simulink model "Oving4Oppg5b"  (R2020b)
settings: Solver=VariableStepAuto  StartTime=0.0  StopTime=130  MaxStep=0.01  RelTol=1e-3
values from neighbouring files (symbols this model uses):
  A = 2.34    [Oving4Oppg5Variables.mat]
  C_d = 0.24    [Oving4Oppg5Variables.mat]
  d = -3696.57031172    [Oving4Oppg5Variables.mat]
  k_F = 17.199    [Oving4Oppg5Variables.mat]
  k_P = 4322.801    [Oving4Oppg5Variables.mat]
  m = 2170    [Oving4Oppg5Variables.mat]
  rho = 1.225    [Oving4Oppg5Variables.mat]
  u_0 = -214.9875    [Oving4Oppg5Variables.mat]
  v_0 = 25    [Oving4Oppg5Variables.mat]
settings Model: Creator=crezl  LastModifiedBy=crezl

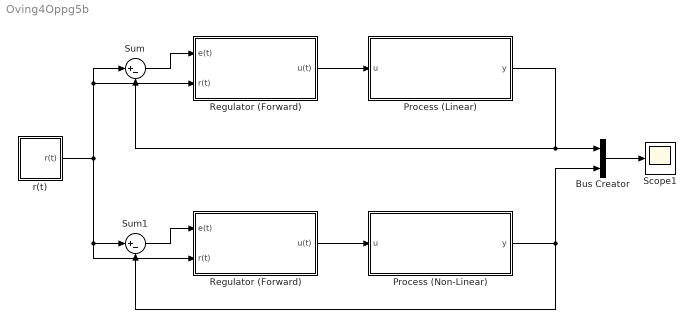
== system Oving4Oppg5b ==
  Bus Creator : BusCreator  Inputs=2
  Process (Linear) : Subsystem
  Process (Non-Linear) : Subsystem
  Regulator (Forward) : Subsystem
  "Regulator (Forward) " : Subsystem
  Scope1 : Scope
  Sum : Sum  Inputs=|+-
  Sum1 : Sum  Inputs=|+-
  r(t) : Subsystem
  wires:
  Process (Linear)/1(y) -> Sum/2, Bus Creator/1
  Bus Creator/1 -> Scope1/1
  Process (Non-Linear)/1(y) -> Bus Creator/2, Sum1/2
  Sum/1 -> Regulator (Forward)/1(e(t))
  r(t)/1(r(t)) -> "Regulator (Forward) "/2(r(t)), Sum1/1, Regulator (Forward)/2(r(t)), Sum/1
  Regulator (Forward)/1(u(t)) -> Process (Linear)/1(u)
  "Regulator (Forward) "/1(u(t)) -> Process (Non-Linear)/1(u)
  Sum1/1 -> "Regulator (Forward) "/1(e(t))

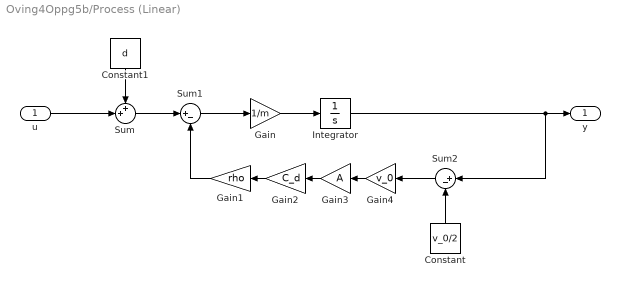
== system Oving4Oppg5b/Process (Linear) ==
  u : Inport
  Constant : Constant  Value=v_0/2
  Constant1 : Constant  Value=d
  Gain : Gain  Gain=1/m
  Gain1 : Gain  Gain=rho
  Gain2 : Gain  Gain=C_d
  Gain3 : Gain  Gain=A
  Gain4 : Gain  Gain=v_0
  Integrator : Integrator  InitialCondition=v_0
  Sum : Sum  Inputs=++|
  Sum1 : Sum  Inputs=|+-
  Sum2 : Sum  Inputs=|+-
  y : Outport
  wires:
  Constant1/1 -> Sum/1
  Integrator/1 -> Sum2/1, y/1
  Sum/1 -> Sum1/1
  Gain1/1 -> Sum1/2
  Sum1/1 -> Gain/1
  Gain3/1 -> Gain2/1
  Gain2/1 -> Gain1/1
  Gain/1 -> Integrator/1
  u/1 -> Sum/2
  Gain4/1 -> Gain3/1
  Constant/1 -> Sum2/2
  Sum2/1 -> Gain4/1

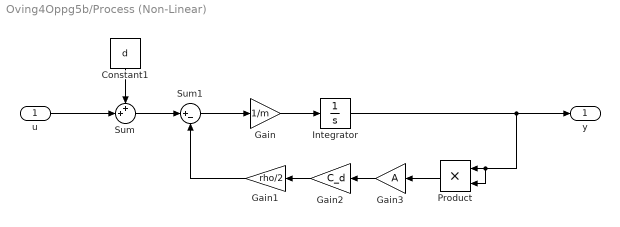
== system Oving4Oppg5b/Process (Non-Linear) ==
  u : Inport
  Constant1 : Constant  Value=d
  Gain : Gain  Gain=1/m
  Gain1 : Gain  Gain=rho/2
  Gain2 : Gain  Gain=C_d
  Gain3 : Gain  Gain=A
  Integrator : Integrator  InitialCondition=v_0
  Product : Product
  Sum : Sum  Inputs=++|
  Sum1 : Sum  Inputs=|+-
  y : Outport
  wires:
  Constant1/1 -> Sum/1
  Integrator/1 -> y/1, Product/2, Product/1
  Sum/1 -> Sum1/1
  Gain1/1 -> Sum1/2
  Sum1/1 -> Gain/1
  Product/1 -> Gain3/1
  Gain3/1 -> Gain2/1
  Gain2/1 -> Gain1/1
  Gain/1 -> Integrator/1
  u/1 -> Sum/2

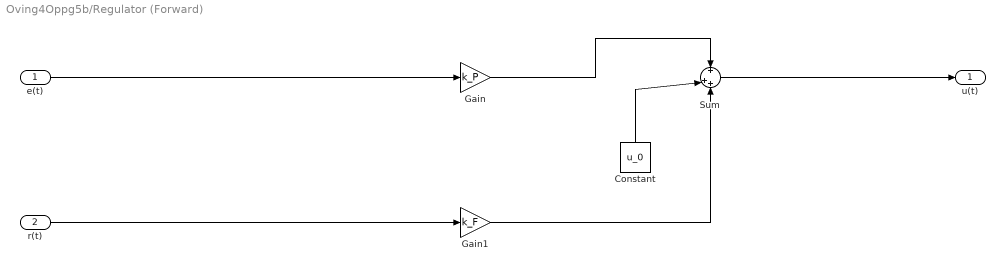
== system Oving4Oppg5b/Regulator (Forward) ==
  e(t) : Inport
  r(t) : Inport  Port=2
  Constant : Constant  Value=u_0
  Gain : Gain  Gain=k_P
  Gain1 : Gain  Gain=k_F
  Sum : Sum  Inputs=+|++
  u(t) : Outport
  wires:
  e(t)/1 -> Gain/1
  Constant/1 -> Sum/2
  Sum/1 -> u(t)/1
  Gain/1 -> Sum/1
  Gain1/1 -> Sum/3
  r(t)/1 -> Gain1/1

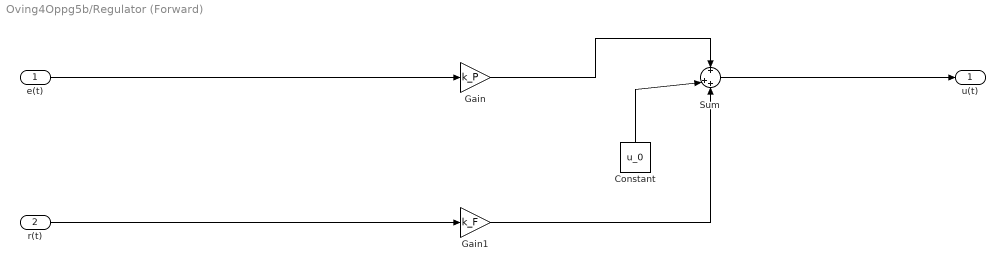
== system Oving4Oppg5b/Regulator (Forward)  ==
  e(t) : Inport
  r(t) : Inport  Port=2
  Constant : Constant  Value=u_0
  Gain : Gain  Gain=k_P
  Gain1 : Gain  Gain=k_F
  Sum : Sum  Inputs=+|++
  u(t) : Outport
  wires:
  e(t)/1 -> Gain/1
  Constant/1 -> Sum/2
  Sum/1 -> u(t)/1
  Gain/1 -> Sum/1
  Gain1/1 -> Sum/3
  r(t)/1 -> Gain1/1

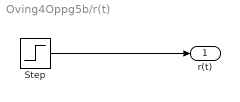
== system Oving4Oppg5b/r(t) ==
  Step : Step  Time=60  Before=25  After=40  SampleTime=0
  r(t) : Outport
  wires:
  Step/1 -> r(t)/1
